simulink model "math_function"  (R2024b)
settings: Solver=VariableStepAuto  StartTime=0.0  StopTime=10.0  RelTol=1e-3
values from neighbouring files (symbols this model uses):
  A = 1.7    [parameters.m]
settings Model: Creator=kavin  LastModifiedBy=kavin

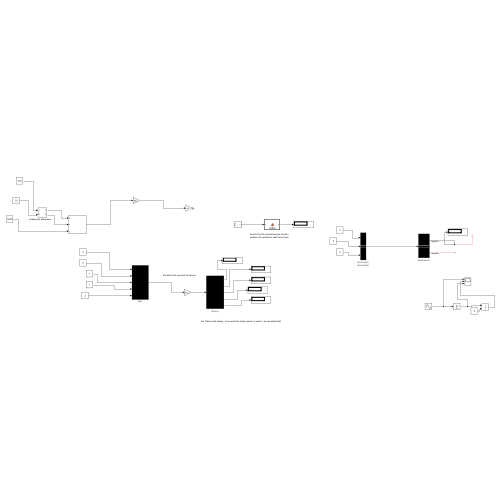
[thumbnail: Simulink's stored preview of the top-level diagram]
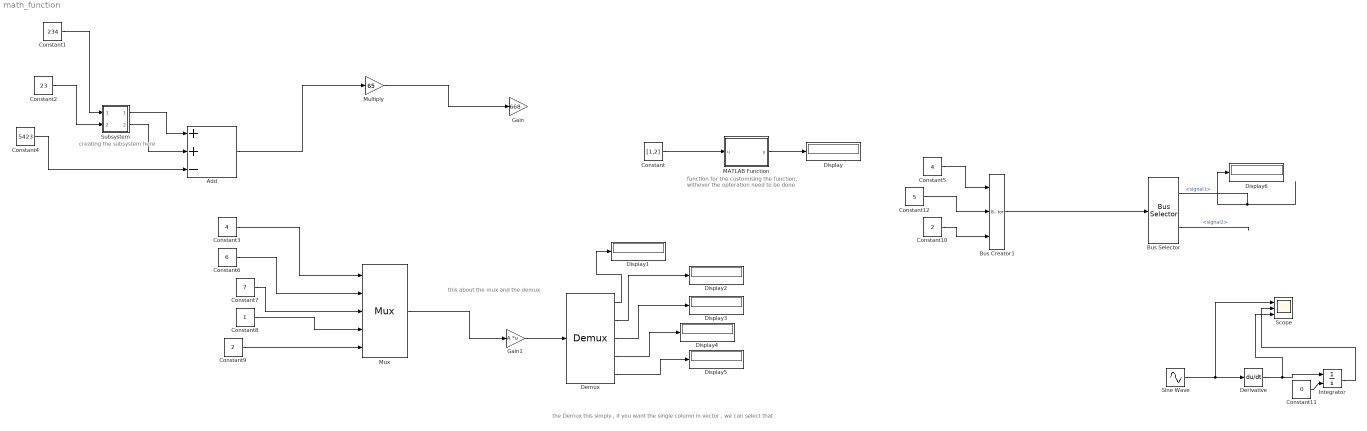
== system math_function ==
  note: the Demux this simply , it you want the single column in vector , we can select that
  note: this about the mux and the demux
  note: creating the subsystem here
  note: function for the customising the function, withever the opteration need to be done
  Add : Sum  Inputs=++-
  Bus Creator1 : BusCreator  Inputs=3
      settings: AttributesFormatString=|
      | %<BlockType>
      | %<BlockType>
  Bus Selector : BusSelector  OutputSignals=signal1,signal2
      settings: AttributesFormatString=%<BlockType>
  Constant : Constant  Value=[1,2]
  Constant1 : Constant  Value=234
  Constant10 : Constant  Value=2
  Constant11 : Constant  Value=0
  Constant12 : Constant  Value=5
  Constant2 : Constant  Value=23
  Constant3 : Constant  Value=4
  Constant4 : Constant  Value=5423
  Constant5 : Constant  Value=4
  Constant6 : Constant  Value=6
  Constant7 : Constant  Value=7
  Constant8 : Constant
  Constant9 : Constant  Value=2
  Demux : Demux  Outputs=5
      settings: AttributesFormatString=%<BlockType>
  Derivative : Derivative
  Display{,1..6} (7 alike) : Display
  Gain : Gain  Gain=668
  Gain1 : Gain  Gain=A  Multiplication=Matrix(K*u)
  Integrator : Integrator  InitialConditionSource=external
  MATLAB Function : MATLAB Function  TreatAsAtomicUnit=on
  Multiply : Gain  Gain=65
  Mux : Mux  Inputs=5
      settings: AttributesFormatString=%<BlockType>
  Scope : Scope  NumInputPorts=3
  Sine Wave : Sin  Frequency=2*pi  SampleTime=0
  Subsystem : Subsystem
  wires:
  Add/1 -> Multiply/1
  Constant/1 -> MATLAB Function/1(u)
  MATLAB Function/1(y) -> Display/1
  Constant4/1 -> Add/3
  Multiply/1 -> Gain/1
  Constant1/1 -> Subsystem/1(In1)
  Constant2/1 -> Subsystem/2(In2)
  Subsystem/1(Out1) -> Add/1
  Subsystem/2(Out2) -> Add/2
  Demux/2 -> Display2/1
  Constant3/1 -> Mux/1
  Constant6/1 -> Mux/2
  Constant7/1 -> Mux/3
  Constant8/1 -> Mux/4
  Constant9/1 -> Mux/5
  Gain1/1 -> Demux/1
  Mux/1 -> Gain1/1
  Demux/1 -> Display1/1
  Demux/3 -> Display3/1
  Demux/4 -> Display4/1
  Demux/5 -> Display5/1
  Constant12/1 -> Bus Creator1/2
  Constant10/1 -> Bus Creator1/3
  Constant5/1 -> Bus Creator1/1
  Bus Creator1/1 -> Bus Selector/1
  Bus Selector/1 -> Display6/1  "<signal1>"
  Bus Selector/2 -> ?  "<signal2>"
  Sine Wave/1 -> Scope/1, Derivative/1
  Derivative/1 -> Scope/3, Integrator/1
  Integrator/1 -> Scope/2
  Constant11/1 -> Integrator/2

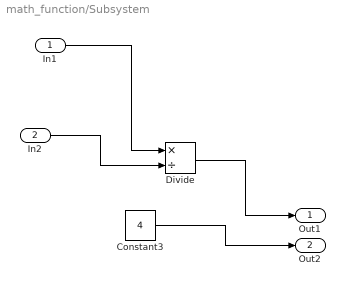
== system math_function/Subsystem ==
  In1 : Inport
  In2 : Inport  Port=2
  Constant3 : Constant  Value=4
  Divide : Product  Inputs=*/
  Out1 : Outport
  Out2 : Outport  Port=2
  wires:
  Divide/1 -> Out1/1
  Constant3/1 -> Out2/1
  In1/1 -> Divide/1
  In2/1 -> Divide/2

== matlab function math_function/MATLAB Function ==
  data: u input; y output
function y =myabs(u)
a=u.^2;
b=sum(a);
y= sqrt(b);
